simulink model "mfcFastStep"  (R2015a)
settings: Solver=ode15s  StartTime=0.0  StopTime=.5  RelTol=1e-6  AbsTol=1e-9
InitFcn:
  | delta = 20;
  | kmu = 20000;
  | 
  | beta = 0;
  | %beta = -10;
  | gamma = 0;
  | gamma = 5;
  | 
  | dummy = 0;
  | 
  | %mfcInit = [5.726117682433310 0.030299840936202];
  | mfcInit = [2.669576823097345 0.018077651410068];
libraries: powerlib_meascontrol x1
settings Model: Creator=ironi  LastModifiedBy=ironi
settings HardwareCC: ProdBitPerLong=64  ProdBitPerPointer=64  ProdWordSize=64  ProdHWDeviceType=Generic->64-bit Embedded Processor (LP64)

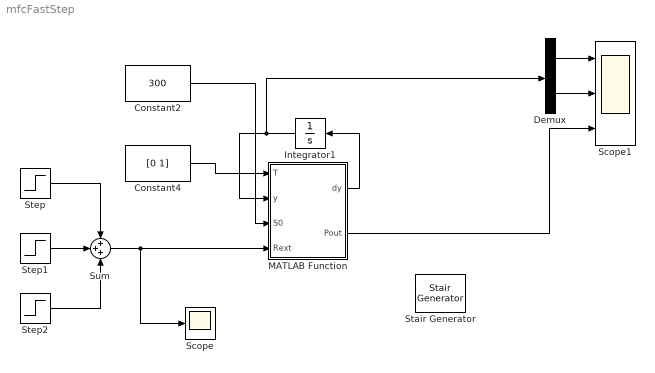
== system mfcFastStep ==
  Constant2 : Constant  Value=300
  Constant4 : Constant  Value=[0 1]
  Demux : Demux  Outputs=2
  Integrator1 : Integrator  InitialCondition=mfcInit
  MATLAB Function : MATLAB Function  TreatAsAtomicUnit=on
  Scope : Scope
  Scope1 : Scope  NumInputPorts=3
      settings: YMin=-5~-5~-5  YMax=5~5~5  SaveName=data
  Stair Generator : powerlib_meascontrol/Pulse & Signal Generators/Stair Generator  t=[0, 1, 3, 3.5]  e=[1, -1, 2.5, 0]  Ts=0
  Step : Step  Time=0  After=200  SampleTime=0
  Step1 : Step  Time=.1  SampleTime=0
  Step2 : Step  Time=4000  After=0  SampleTime=0
  Sum : Sum  Inputs=+++
  wires:
  MATLAB Function/1(dy) -> Integrator1/1
  Integrator1/1 -> Demux/1, MATLAB Function/2(y)
  Constant4/1 -> MATLAB Function/1(T)
  Constant2/1 -> MATLAB Function/3(S0)
  Demux/2 -> Scope1/2
  Demux/1 -> Scope1/1
  MATLAB Function/2(Pout) -> Scope1/3
  Step/1 -> Sum/1
  Step1/1 -> Sum/2
  Step2/1 -> Sum/3
  Sum/1 -> MATLAB Function/4(Rext), Scope/1

== matlab function mfcFastStep/MATLAB Function ==
  data: T input; dy output; y input; dummy parameter; S0 input; Rext input; Pout output
function [dy, Pout]= mfcModelFast(T, y, dummy, S0, Rext)
F = 96485;%
R = 8.314472;%
T = 298.15;%
yield = 22.753;%
% Ych4 = .3;%
qmax_a = 8.484;%
qmax_m = 8.2;%
umax_a = 1.9753;%
umax_m = .1;%
Ks_a = 20;%
Ks_m = 80;%
m = 2;%
gamma = 663400;%
Mtotal = .05;%
Km = .2*Mtotal;%
% Kd_a = .02*umax_a;%
% Kd_m = .02*umax_m;%
Xmax = 512.5;%
Kx = .01*4;%
Rmin = 25;%
Rmax = 2000 + Rmin;%
Emin = .01;%
Emax = 0.25 + 0.4144+ Emin;%
Kr = .024;%

% i0ref=0.4*4;%

e = 0.0001*Mtotal;%

V = 0.2;%
Fin = 0.1527;%

D = Fin/V;

Xtot = 500;

Xeg = 250;

S   = y(1);
Mox = y(2);
xm = Xtot - Xeg;


%% Équations dynamiques
  
Mred = Mtotal - Mox;

Rint = Rmin + (Rmax - Rmin) * exp(-Kr*Xeg);                         % (22)
Eocv = Emin + (Emax - Emin) * exp(-1/(Kr*Xeg));                     % (23)

% alpha = 1/2*(1 + tanh(Kx*(Xeg + xm - Xmax)));                    % (9)

qa = qmax_a * S / (Ks_a + S) * Mox / (Km + Mox);                    % (15)
qm = qmax_m * S / (Ks_m + S);                                       % (16)

% ueg = umax_a * S / (Ks_a + S) * Mox / (Km + Mox);                    % (13)

% Imfc = (Eocv - n_conc) / (Rext + Rint) * Mred / (e + Mred);         % (21)
temp = Eocv - (R*T/m/F)*abs(log(complex(Mtotal/Mred)));
% Imfc = (Eocv - (R*T/m/F)*abs(log(complex(Mtotal/Mred))))/(Rext+Rint)*Mred/(e+Mred);
Imfc = temp/(Rext+Rint)*Mred/(e+Mred);

% Pout = ((Eocv - (R*T/m/F)*abs(log(complex(Mtotal/Mred))))*Mred/(e+Mred)-Rint*Imfc)*Imfc;
Pout = (temp*Mred/(e+Mred)-Rint*Imfc)*Imfc;

Sp = -qa*Xeg - qm*xm + D*(S0 - S);                                   % (6)
% Xap = ueg*xa - Kd_a*xa - alpha_a*D*xa;                               % (7)
% Xmp = um*xm - Kd_m*xm - alpha_m*D*xm;                               % (8)

Moxp = -yield*qa + gamma*Imfc / (m*F*V*Xeg) * 86400;                 % (12)

% if xa < 1 && Xap < 0
%   Xap = 0;
% end
% 
% if xm < 0.99 && Xmp < 0
%   Xmp = 0;
% end

% Pout = Rext*Imfc^2;

% dy = [Sp; Xap; Xmp; Moxp];
dy = [Sp; Moxp];
